simulink model "Test_VectorIO"  (R2020a)
settings: configuration reference "testConfig" (kept outside this file)
undefined symbols (not defined in the file or in its folder): DiscIntNeverNeededParam
Description:
  | A simple model
settings Model: DataDictionary=TestConfig.sldd  Creator=raarenst  LastModifiedBy=toma
settings ConfigSetRef: SourceName=testConfig

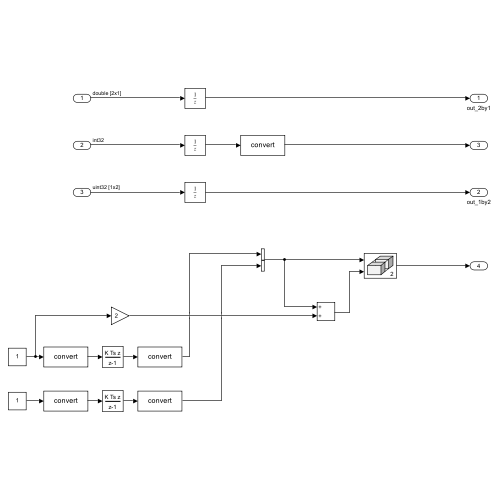
[thumbnail: Simulink's stored preview of the top-level diagram]
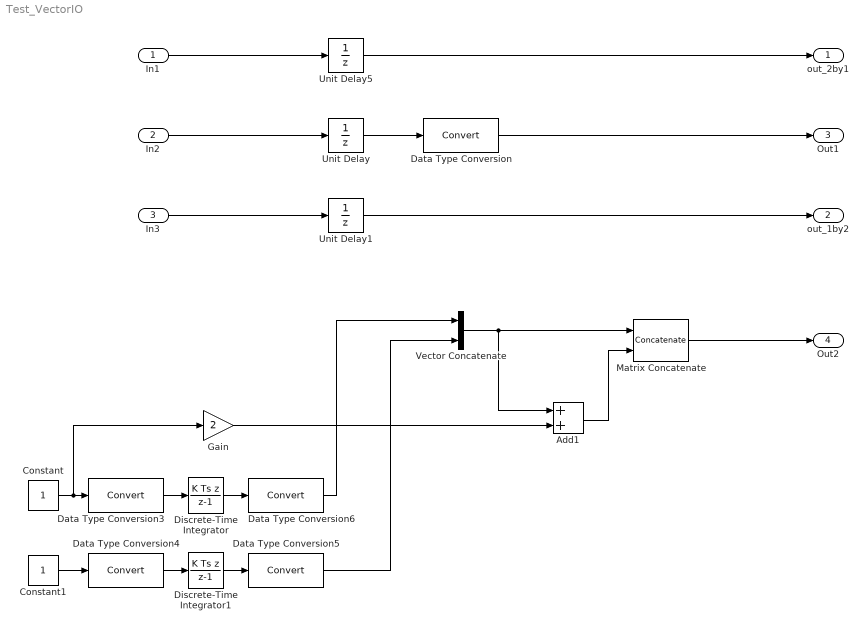
== system Test_VectorIO ==
  In1 : Inport  OutDataTypeStr=double  PortDimensions=[2,1]
  In2 : Inport  Port=2  OutDataTypeStr=int32
  In3 : Inport  Port=3  OutDataTypeStr=uint32  PortDimensions=[1,2]
  Add1 : Sum
  Constant : Constant  OutDataTypeStr=int32  SampleTime=-1
  Constant1 : Constant  OutDataTypeStr=int32  SampleTime=-1
  Data Type Conversion{,3..6} (5 alike) : DataTypeConversion
  Discrete-Time Integrator : DiscreteIntegrator  IntegratorMethod=Integration: Backward Euler  SampleTime=-1  ICPrevOutput=DiscIntNeverNeededParam  ICPrevScaledInput=DiscIntNeverNeededParam
  Discrete-Time Integrator1 : DiscreteIntegrator  IntegratorMethod=Integration: Backward Euler  InitialCondition=1  SampleTime=-1  ICPrevOutput=DiscIntNeverNeededParam  ICPrevScaledInput=DiscIntNeverNeededParam
  Gain : Gain  Gain=2  OutDataTypeStr=int32
  Matrix Concatenate : Concatenate  Mode=Multidimensional array  ConcatenateDimension=2
  Unit Delay : UnitDelay  SampleTime=-1  HasFrameUpgradeWarning=on
  Unit Delay1 : UnitDelay  SampleTime=-1  HasFrameUpgradeWarning=on
  Unit Delay5 : UnitDelay  SampleTime=-1  HasFrameUpgradeWarning=on
  Vector Concatenate : Concatenate
  out_2by1 : Outport
  out_1by2 : Outport  Port=2
  Out1 : Outport  Port=3
  Out2 : Outport  Port=4
  wires:
  In2/1 -> Unit Delay/1
  Unit Delay/1 -> Data Type Conversion/1
  In1/1 -> Unit Delay5/1
  Data Type Conversion/1 -> Out1/1
  Unit Delay1/1 -> out_1by2/1
  In3/1 -> Unit Delay1/1
  Unit Delay5/1 -> out_2by1/1
  Vector Concatenate/1 -> Add1/1, Matrix Concatenate/1
  Discrete-Time Integrator1/1 -> Data Type Conversion5/1
  Discrete-Time Integrator/1 -> Data Type Conversion6/1
  Constant/1 -> Gain/1, Data Type Conversion3/1
  Data Type Conversion3/1 -> Discrete-Time Integrator/1
  Data Type Conversion4/1 -> Discrete-Time Integrator1/1
  Data Type Conversion5/1 -> Vector Concatenate/2
  Data Type Conversion6/1 -> Vector Concatenate/1
  Constant1/1 -> Data Type Conversion4/1
  Add1/1 -> Matrix Concatenate/2
  Matrix Concatenate/1 -> Out2/1
  Gain/1 -> Add1/2
